simulink library "lasPosEst_cl"  (R2020a)
settings: Solver=VariableStepAuto  StartTime=0.0  StopTime=10.0  RelTol=1e-3
undefined symbols (not defined in the file or in its folder): initializeBussesFromBlock
libraries: lineAngleSensor x1
settings Model: Creator=mcobb  LastModifiedBy=andre
settings DataIOCC: ReturnWorkspaceOutputs=off
settings DebuggingCC: ArithmeticOperatorsInVariantConditions=warning
settings SFSimCC: CustomCodeUndefinedFunction=UseInterfaceOnly

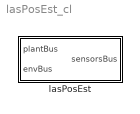
== system lasPosEst_cl ==
  lasPosEst : Subsystem  LoadFcn=initializeBussesFromBlock(gcb)  InitFcn=initializeBussesFromBlock(gcb)  StartFcn=initializeBussesFromBlock(gcb)  VariantControl=VSS_sensors_realisticSensors

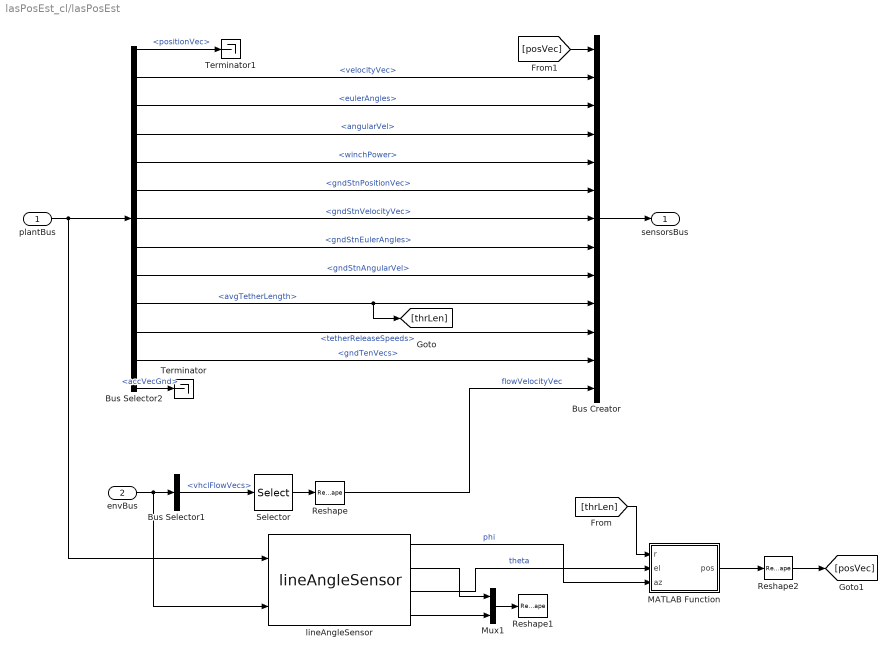
== system lasPosEst_cl/lasPosEst ==
  plantBus : Inport  OutDataTypeStr=Bus: plantBus
  envBus : Inport  Port=2  OutDataTypeStr=Bus: envBus
  Bus Creator : BusCreator  Inputs=13  OutDataTypeStr=Bus: sensorsBus  NonVirtualBus=on
      settings: InheritFromInputs=off
  Bus Selector1 : BusSelector  OutputSignals=vhclFlowVecs
  Bus Selector2 : BusSelector  OutputSignals=positionVec,velocityVec,eulerAngles,angularVel,winchPower,gndStnPositionVec,gndStnVelocityVec,gndStnEulerAngles,gndStnAngularVel,avgTetherLength,tetherReleaseSpeeds,gndTenVecs,accVecGnd
  MATLAB Function : MATLAB Function  TreatAsAtomicUnit=on
  Mux1 : Mux  Inputs=2
  Reshape : Reshape  OutputDimensionality=Column vector (2-D)
  Reshape1 : Reshape  OutputDimensionality=Column vector (2-D)
  Reshape2 : Reshape  OutputDimensionality=Column vector (2-D)
  Selector : Selector  NumberOfDimensions=2  InputPortWidth=3  IndexOptions=Select all,Index vector (dialog)  Indices=[1 3],1  OutputSizes=1,1
  Terminator : Terminator
  Terminator1 : Terminator
  lineAngleSensor : lineAngleSensor/lineAngleSensor  las=las  env=env
  sensorsBus : Outport  OutDataTypeStr=Bus: sensorsBus  VectorParamsAs1DForOutWhenUnconnected=off
  wires:
  Bus Selector2/8 -> Bus Creator/8  "<gndStnEulerAngles>"
  Bus Selector2/4 -> Bus Creator/4  "<angularVel>"
  Bus Selector2/3 -> Bus Creator/3  "<eulerAngles>"
  Bus Selector2/9 -> Bus Creator/9  "<gndStnAngularVel>"
  Bus Creator/1 -> sensorsBus/1
  Bus Selector2/12 -> Bus Creator/12  "<gndTenVecs>"
  Bus Selector2/7 -> Bus Creator/7  "<gndStnVelocityVec>"
  Bus Selector2/10 -> [thrLen], Bus Creator/10  "<avgTetherLength>"
  Bus Selector2/11 -> Bus Creator/11  "<tetherReleaseSpeeds>"
  envBus/1 -> Bus Selector1/1, lineAngleSensor/2
  Mux1/1 -> Reshape1/1
  lineAngleSensor/3 -> MATLAB Function/2(el)  "theta"
  Selector/1 -> Reshape/1
  Bus Selector2/2 -> Bus Creator/2  "<velocityVec>"
  lineAngleSensor/4 -> Mux1/2
  lineAngleSensor/2 -> Mux1/1
  lineAngleSensor/1 -> MATLAB Function/3(az)  "phi"
  Bus Selector2/5 -> Bus Creator/5  "<winchPower>"
  plantBus/1 -> lineAngleSensor/1, Bus Selector2/1
  Bus Selector2/1 -> Terminator1/1  "<positionVec>"
  Bus Selector1/1 -> Selector/1  "<vhclFlowVecs>"
  Reshape/1 -> Bus Creator/13  "flowVelocityVec"
  Bus Selector2/6 -> Bus Creator/6  "<gndStnPositionVec>"
  Bus Selector2/13 -> Terminator/1  "<accVecGnd>"
  [thrLen] -> MATLAB Function/1(r)
  MATLAB Function/1(pos) -> Reshape2/1
  Reshape2/1 -> [posVec]
  [posVec] -> Bus Creator/1

== matlab function lasPosEst_cl/lasPosEst/MATLAB Function ==
  data: r input; pos output; el input; az input
function pos = fcn(r,el,az)

x = -r .* cos(el) .* cos(az)
y = r .* cos(el) .* sin(az)
z = r .* sin(el);
pos = [x y z];
